simulink model "MPPT_SimulationSetup"  (Simulink 10.1)
settings: Solver=ode23tb  StartTime=0.0  StopTime=0.5  RelTol=1e-3  EnableMultiTasking=on
libraries: powerlib x13, simulink x1
settings Model: Creator=XUAN TRUONG  LastModifiedBy=vishn
settings DataIOCC: LimitDataPoints=on  SignalLoggingSaveFormat=ModelDataLogs
settings OptimizationCC: ExpressionDepthLimit=2147483647
settings DebuggingCC: SolverPrmCheckMsg=warning  FcnCallInpInsideContextMsg=warning  StateNameClashWarn=warning

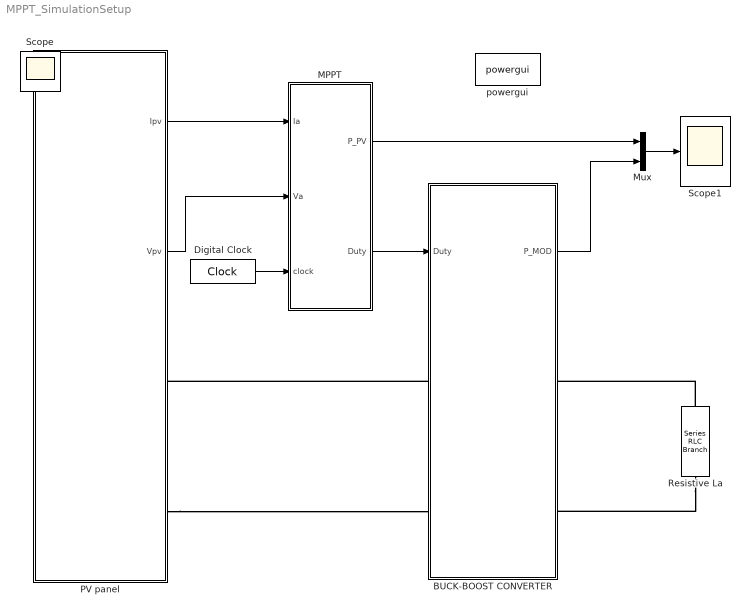
== system MPPT_SimulationSetup ==
  BUCK-BOOST CONVERTER : Subsystem
  Digital Clock : DigitalClock  SampleTime=0.001
  MPPT : Subsystem
  Mux : Mux  Inputs=2
  PV panel : Subsystem
  Resistive La : powerlib/Elements/Series RLC Branch  LConnTagsString=__new0  RConnTagsString=__new0  BranchType=R  Resistance=30  Inductance=1e-3  SetiL0=off  InitialCurrent=0  Capacitance=1e-6  Setx0=off  InitialVoltage=0  Measurements=None
  Scope1 : Scope
  powergui : powerlib/powergui  SimulationMode=Discrete  SolverType=Tustin  SampleTime=1e-6  frequency=60  SPID=off  DisableSnubberDevices=off  DisableRonSwitches=off  DisableVfSwitches=off  SwTol=0  Interpol=off  DisplayEquations=off  FunctionMessages=off  frequencyindice=0  Pbase=100e6  ErrMax=1e-4  Iterations=50  UnitsV=kV  UnitsW=MW  echomessages=off  HookPort=off  EnableUseOfTLC=off  x0status=blocks  RestoreLinks=warning  ResistiveCurrentMeasurement=off  Frange=[0:2:500]  Ylog=off  Xlog=on  ShowGrid=off  save=off  variable=ZData  structure=ScopeData  ZoomFFT=off  StartTime=0.04  cycles=2  DisplayStyle=1  fundamental=1000  FreqAxis=off  MaxFrequency=50000  frequencyindicesteady=1  RmsSteady=1  display=off  Ts=0  methode=off
  Scope : Scope
  wires:
  PV panel/1(Ipv) -> MPPT/1(Ia)
  PV panel/2(Vpv) -> MPPT/2(Va)
  Digital Clock/1 -> MPPT/3(clock)
  MPPT/2(Duty) -> BUCK-BOOST CONVERTER/1(Duty)
  MPPT/1(P_PV) -> Mux/1
  BUCK-BOOST CONVERTER/1(P_MOD) -> Mux/2
  Mux/1 -> Scope1/1
  connections:
  Resistive La/RConn1 -- BUCK-BOOST CONVERTER/RConn2
  PV panel/RConn2 -- BUCK-BOOST CONVERTER/LConn2
  Resistive La/LConn1 -- BUCK-BOOST CONVERTER/RConn1
  BUCK-BOOST CONVERTER/LConn1 -- PV panel/RConn1

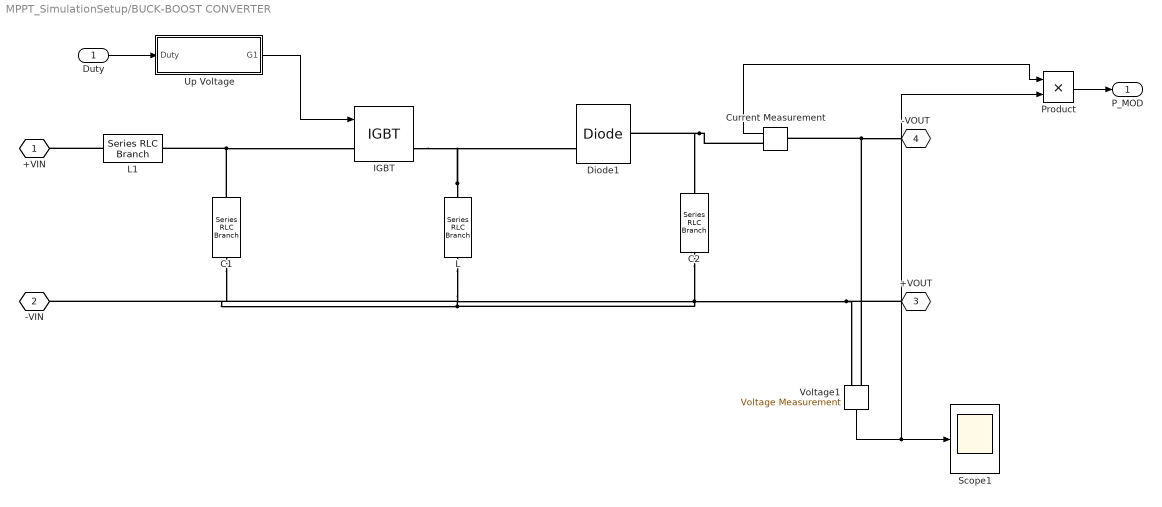
== system MPPT_SimulationSetup/BUCK-BOOST CONVERTER ==
  Duty : Inport
  " C1" : powerlib/Elements/Series RLC Branch  LConnTagsString=__new0  RConnTagsString=__new0  BranchType=C  Resistance=5  Inductance=0.05  SetiL0=off  InitialCurrent=0  Capacitance=2000e-6  Setx0=on  InitialVoltage=0  Measurements=Branch voltage and current
  " C2" : powerlib/Elements/Series RLC Branch  LConnTagsString=__new0  RConnTagsString=__new0  BranchType=C  Resistance=5  Inductance=0.05  SetiL0=off  InitialCurrent=0  Capacitance=2000e-6  Setx0=on  InitialVoltage=0  Measurements=Branch voltage and current
  " L" : powerlib/Elements/Series RLC Branch  LConnTagsString=__new0  RConnTagsString=__new0  BranchType=L  Resistance=5  Inductance=47e-6  SetiL0=on  InitialCurrent=0  Capacitance=1.0  Setx0=off  InitialVoltage=0  Measurements=Branch voltage and current
  " L1" : powerlib/Elements/Series RLC Branch  LConnTagsString=__new0  RConnTagsString=__new0  BranchType=L  Resistance=5  Inductance=1000e-6  SetiL0=on  InitialCurrent=0  Capacitance=1.0  Setx0=off  InitialVoltage=0  Measurements=Branch voltage and current
  Current Measurement : powerlib/Measurements/Current Measurement  PhasorSimulation=off  OutputType=Complex  PSBequivalent=0
  Diode1 : powerlib/Power Electronics/Diode  Ron=0.00001  Lon=0  Vf=0.8  IC=0  UseSnubber=off  Rs=1e4  Cs=1e-4  Measurements=on
  IGBT : powerlib/Power Electronics/IGBT  Ron=0.00001  Lon=0  Vf=2.5  Tf=1e-6  Tt=1e4  IC=0  Rs=1e5  Cs=inf  Measurements=on
  Product : Product  RndMeth=Zero
  Scope1 : Scope
  Up Voltage : Subsystem  mask{fc=10000, Gama=0.5}
      mask prompts: fc "Frequency (Hz)"; Gama "Duty Cycle  (0-1)"
      mask Display: disp('CONTROL SIGNAL')
  Voltage1 : powerlib/Measurements/Voltage Measurement  PhasorSimulation=off  OutputType=Complex  PSBequivalent=0
  +VIN : PMIOPort  Tag=PMCPort  Side=Left
  -VIN : PMIOPort  Tag=PMCPort  Port=2  Side=Left
  +VOUT : PMIOPort  Tag=PMCPort  Port=3  Side=Right
  -VOUT : PMIOPort  Tag=PMCPort  Port=4  Side=Right
  P_MOD : Outport
  wires:
  Voltage1/1 -> Scope1/1, Product/2
  Duty/1 -> Up Voltage/1(Duty)
  Up Voltage/1(G1) -> IGBT/1
  Current Measurement/1 -> Product/1
  Product/1 -> P_MOD/1
  connections:
  Voltage1/LConn2 -- -VOUT/RConn1 -- Current Measurement/LConn1
  " L"/RConn1 -- -VIN/RConn1 -- " C1"/RConn1 -- +VOUT/RConn1 -- Voltage1/LConn1 -- " C2"/RConn1
  " L"/LConn1 -- IGBT/RConn1 -- Diode1/RConn1
  " C1"/LConn1 -- IGBT/LConn1 -- " L1"/LConn1
  Current Measurement/RConn1 -- Diode1/LConn1 -- " C2"/LConn1
  " L1"/RConn1 -- +VIN/RConn1

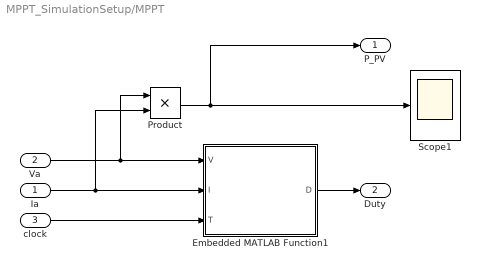
== system MPPT_SimulationSetup/MPPT ==
  Ia : Inport
  Va : Inport  Port=2
  clock : Inport  Port=3
  Embedded MATLAB Function1 : MATLAB Function  TreatAsAtomicUnit=on
  Product : Product  RndMeth=Zero
  Scope1 : Scope
  P_PV : Outport
  Duty : Outport  Port=2
  wires:
  Ia/1 -> Product/2, Embedded MATLAB Function1/2(I)
  Va/1 -> Product/1, Embedded MATLAB Function1/1(V)
  clock/1 -> Embedded MATLAB Function1/3(T)
  Product/1 -> Scope1/1, P_PV/1
  Embedded MATLAB Function1/1(D) -> Duty/1

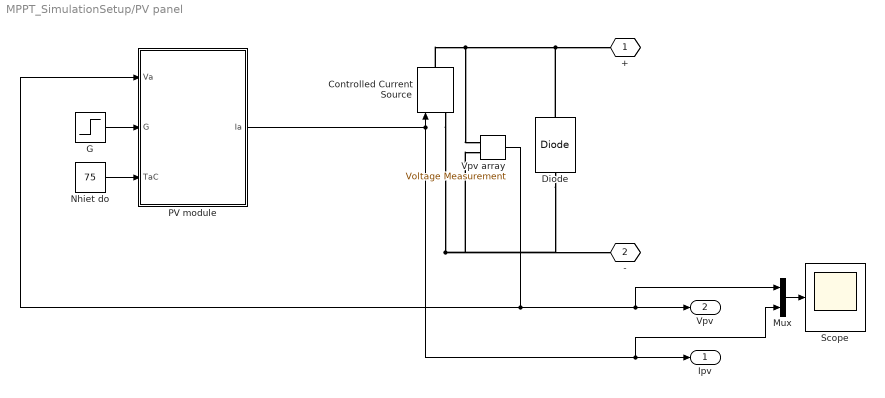
== system MPPT_SimulationSetup/PV panel ==
  Controlled Current Source : powerlib/Electrical Sources/Controlled Current Source  Initialize=on  Source_Type=AC  Amplitude=0  Phase=0  Frequency=0  Measurements=None
  Diode : powerlib/Power Electronics/Diode  Ron=0.001  Lon=0  Vf=0  IC=0  UseSnubber=off  Rs=500  Cs=250e-9  Measurements=off
  G : Step  Time=0  SampleTime=0
  Mux : Mux  Inputs=2
  Nhiet do : Constant  Value=75
  PV module : MATLAB Function  TreatAsAtomicUnit=on
  Scope : Scope
  Vpv array : powerlib/Measurements/Voltage Measurement  PhasorSimulation=off  OutputType=Complex  PSBequivalent=0
  + : PMIOPort  Tag=PMCPort  Side=Right
  - : PMIOPort  Tag=PMCPort  Port=2  Side=Right
  Ipv : Outport
  Vpv : Outport  Port=2
  wires:
  G/1 -> PV module/2(G)
  Nhiet do/1 -> PV module/3(TaC)
  PV module/1(Ia) -> Controlled Current Source/1, Ipv/1, Mux/2
  Vpv array/1 -> PV module/1(Va), Vpv/1, Mux/1
  Mux/1 -> Scope/1
  connections:
  Controlled Current Source/LConn1 -- Diode/LConn1 -- -/RConn1 -- Vpv array/LConn2
  Controlled Current Source/RConn1 -- Diode/RConn1 -- +/RConn1 -- Vpv array/LConn1

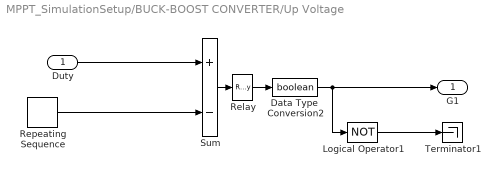
== system MPPT_SimulationSetup/BUCK-BOOST CONVERTER/Up Voltage ==
  Duty : Inport
  Data Type  Conversion2 : DataTypeConversion  OutDataTypeStr=boolean  SaturateOnIntegerOverflow=on  RndMeth=Zero
  Logical Operator1 : Logic  Operator=NOT
  Relay : Relay
  Repeating Sequence : simulink/Sources/Repeating Sequence  rep_seq_t=[0 1/10e3]  rep_seq_y=[0 1]
  Sum : Sum  Inputs=+-  InputSameDT=on  SaturateOnIntegerOverflow=on  OutDataTypeStr=Inherit: Same as first input
  Terminator1 : Terminator
  G1 : Outport
  wires:
  Data Type  Conversion2/1 -> Logical Operator1/1, G1/1
  Duty/1 -> Sum/1
  Repeating Sequence/1 -> Sum/2
  Sum/1 -> Relay/1
  Relay/1 -> Data Type  Conversion2/1
  Logical Operator1/1 -> Terminator1/1

== matlab function MPPT/Embedded MATLAB Function1 ==
  data: V input double; I input double; T input double; D output double
function D   = ACO(V,I,T)
persistent P2  P1  dP d dd n;
if isempty(V)
    V=20;
end
if isempty(I)
    I=0;
end
if isempty(P2)
    P2=0;
end
if isempty(P1)
    P1=0;
end
if isempty(dP)
    dP=0;
end
if isempty(d)
    d=1;
end
if isempty(dd)
    dd=0;
end
if isempty(n)
    n=1;
end
%%%%%%%%%%%%%%%%%%%%%
    if  (T > n*0.02)   %chu ki lay mau 0.02s
    n = n + 1;
    P1=P2;
    P2=V*I;
    dP=P2-P1;
    if (dd==0)
        if dP>1
            dd=0.01;
            d=d+dd;
        else
            if dP<-1
                dd=-0.01;
                d=d+dd;
            else
                dd=0;
            end
        end
    else
        if ((dP<1)&&(dP>-1))
        dd=0;
        d=d+dd;
        else
            if ((dP/dd)>0)
                dd=0.01;
                d=d+dd;
            else
                dd=-0.01;
                d=d+dd;
            end
        end
    end    
    end
D=d/(d+1);
if D<0.1
    D=0.1;
    d=D/(1-D);
else
    if D>0.9
        D=0.9;
        d=D/(1-D);
    else
    end
end
end

== matlab function PV panel/PV module ==
  data: Va input double; Ia output double; G input double; TaC input double
function Ia=Iphoton(Va,G,TaC) 
% Cac tham so lay tu bo pin mat troi Kyocera KC50T PER labs - HCMUT
% Ham tinh toan dong ra pin duoi su thay doi nhiet do va do roi 
% Out: Ia = Module operating current (A)
% In:  Va = Module operating voltage (V)
%      G = Do roi (1G = 1000 W/m^2)
%      TaC = Nhiet do module(celsius)
% rewrite by Xuan Truong – Hoai Phong 25-12-2011
% Falcuty of Ho Chi Minh City University of Technology 
% Director : PD . Le Minh Phuong 
% Falcuty of Ho Chi Minh City University of Technolo
%----------------------------------------------------------------------
k = 1.381e-23;      % hang so Boltzmann  
q = 1.602e-19;      % dien tich electron 
n = 1.3;           % hang so diode ly tuong (1<n<2)
Eg = 1.12;          % Nang luong khe; 1.12eV (Si), 1.42 (GaAs) 
Ns = 10;            % so cell 
Np=6;
TrK = 298;          %25 do C
Voc_TrK = 37.51 /Ns; % Voc : Ap ho mach 25 do C 
Isc_TrK = 8.63/Np;     % Isc: dong dien ngan mach tham khao o 25 do C                                             
a = 1.33e-3;        % He so tang dong theo nhiet do (0.065A/C) 
TaK = 273 + TaC;     % Nhiet do module thi nghiem
Vc = Va / Ns;       % Ap tren tung cell 
% Dong ngan mach thi nghiem
Isc = Isc_TrK * (1 + (a * (TaK - TrK))); 
% Dong photon phat ra o do roi G(thong thuong G=1KW/m2)
Iph = G * Isc;  
% The nhiet tai 25 do C 
Vt_TrK = n * k * TrK / q;    
% Goi b = Eg * q/(n*k) 
b = Eg * q /(n * k); 
% Tinh toan dong bao hoa Io 
Ir_TrK = Isc_TrK / (exp(Voc_TrK / Vt_TrK) -1); 
Ir = Ir_TrK * (TaK / TrK)^(3/n) * exp(-b * (1 / TaK -1 / TrK)); 
% Tinh toan Rs 
dVdI_Voc = -2.0/Ns;    % Take dV/dI @ Voc from I-V curve of datasheet 
Xv = Ir_TrK / Vt_TrK * exp(Voc_TrK / Vt_TrK); 
Rs = - dVdI_Voc - 1/Xv;   
% The nhiet thi nghiem 
Vt_Ta = n * k * TaK / q;                                                          
% Ia = Iph - Ir * (exp((Vc + Ia * Rs) / Vt_Ta) -1) 
% f(Ia) = Iph - Ia - Ir * ( exp((Vc + Ia * Rs) / Vt_Ta) -1) = 0 
% Solve for Ia by Newton's method: Ia2 = Ia1 - f(Ia1)/f'(Ia1) 
Ia=zeros(size(Vc)); % Initialize Ia with zeros   
for j=1:5; 
    Ia = Ia - (Iph - Ia - Ir .* ( exp((Vc + Ia .* Rs) ./ Vt_Ta) -1))... 
        ./ (-1 - Ir * (Rs ./ Vt_Ta) .* exp((Vc + Ia .* Rs) ./ Vt_Ta)); 
end
Ia=Ia*Np;
end
